simulink model "nonlinear_switch_intgr_mgntrqr_wndup_ctrl_closed_loop_sys"  (R2020b)
settings: Solver=VariableStepAuto  StartTime=0.0  StopTime=800  RelTol=1e-3
values from neighbouring files (symbols this model uses):
  COMMANDED_TORQUE_SATURATION = 0.05    [Workshop_MATLAB.m]
  COUPLING_COEFFICIENT = 0.5736    [Workshop_MATLAB.m]
  DEADZONE_REACTION_WHEEL_ANGULAR_MOMENTUM = REACTION_WHEEL_INERTIA * DEADZONE_REACTION_WHEEL_VELOCITY * dcgain(REACTION_WHEEL_ANGULAR_MOMENTUM.TRANSFER_FUNCTION)    [Workshop_MATLAB.m]
  deadzoneControllerGain = 0.1    [Workshop_MATLAB.m]
  DISTURBANCE_TORQUE = 0.001    [Workshop_MATLAB.m]
  DISTURBANCE_TORQUE_DELAY = 100    [Workshop_MATLAB.m]
  ESTIMATOR_TRANSFER_FUNCTION_DENOMINATOR = [ESTIMATOR_TIME_CONSTANT 1]    [Workshop_MATLAB.m]
  ESTIMATOR_TRANSFER_FUNCTION_NUMERATOR = [1 0]    [Workshop_MATLAB.m]
  FLEXIBLE_MODE_DAMPING_RATIO = 0.00495    [Workshop_MATLAB.m]
  FLEXIBLE_MODE_FREQUENCY = 2.6268    [Workshop_MATLAB.m]
  INITIAL_CONDITION_ON_STATE = 0.0001    [Workshop_MATLAB.m]
  MAGNETORQUER_CONTROLLER_GAIN = 0.001    [Workshop_MATLAB.m]
  MAXIMUM_LARGE_POINTING_ERROR = 25*2*pi/360    (= 0.436332312999)    [Workshop_MATLAB.m]
  MAXIMUM_TOLERABLE_POINTING_ERROR = 2.7*2*pi/360    (= 0.0471238898038)    [Workshop_MATLAB.m]
  MEASUREMENT_DELAY = 0.8    [Workshop_MATLAB.m]
  MEASUREMENT_NOISE_VARIANCE = 10^(-9)    (= 1e-09)    [Workshop_MATLAB.m]
  modalWithIntegratorGainMatrixStateFeedback = [0.0223 -0.55 -5.7]    [Workshop_MATLAB.m]
  NON_LINEAR_CONTROL_GAIN = 6    [Workshop_MATLAB.m]
  NON_LINEAR_CONTROL_SPEED_COMMAND = 0.15*pi/180    (= 0.00261799387799)    [Workshop_MATLAB.m]
  NON_LINEAR_CONTROL_SWITCHING_THRESHOLD = 3*pi/180    (= 0.0523598775598)    [Workshop_MATLAB.m]
  REACTION_WHEEL_DYNAMICS_DENOMINATOR = [1 2.400 0.763]    [Workshop_MATLAB.m]
  REACTION_WHEEL_DYNAMICS_NUMERATOR = REACTION_WHEEL_INERTIA*[1.214 0.763 0]    [Workshop_MATLAB.m]
  REACTION_WHEEL_INERTIA = 0.0004    [Workshop_MATLAB.m]
  REACTION_WHEEL_VELOCITY_SATURATION = 2800*2*pi/60    (= 293.215314335)    [Workshop_MATLAB.m]
  SATELLITE_INERTIA = 31.38    [Workshop_MATLAB.m]
  STAR_TRACKER_NOISE_DELAY = 160    [Workshop_MATLAB.m]
  UNLOADING_TORQUE_SATURATION = 0.0043    [Workshop_MATLAB.m]
undefined symbols (not defined in the file or in its folder): REACTION_WHEEL_ANGULAR_MOMENTUM, sigbuilder_block
libraries: dspsigops x2, simulink x1
settings Model: Creator=WLCG  LastModifiedBy=WLCG

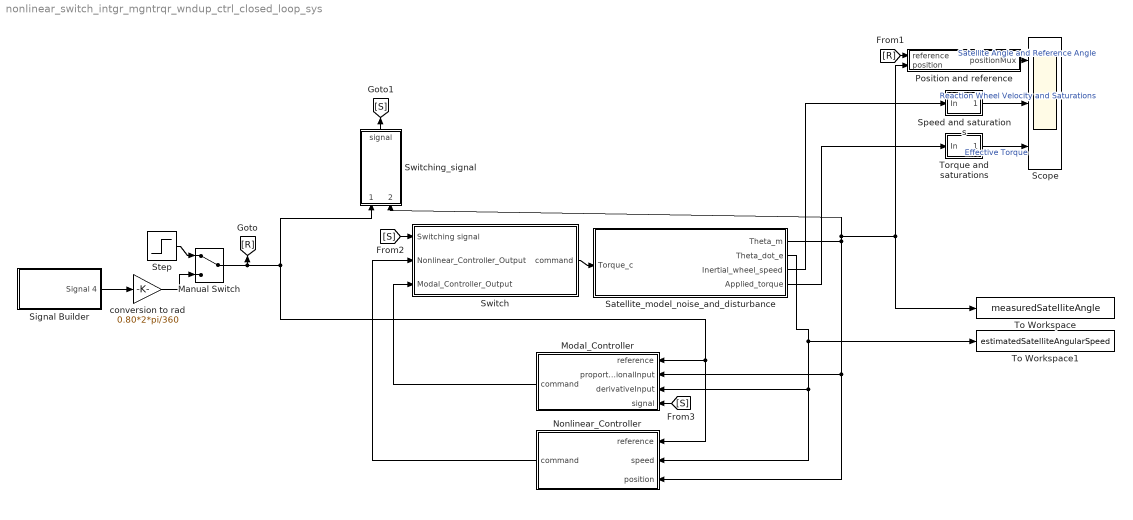
== system nonlinear_switch_intgr_mgntrqr_wndup_ctrl_closed_loop_sys ==
  Manual Switch : ManualSwitch
  Modal_Controller : Subsystem
  Nonlinear_Controller : Subsystem
  Position and reference : Subsystem
  Satellite_model_noise_and_disturbance : Subsystem
  Scope : Scope  NumInputPorts=3
  Signal Builder : Subsystem  Tag=STV Subsys  LoadFcn=sigbuilder_block('load');  StartFcn=sigbuilder_block('start');  StopFcn=sigbuilder_block('stop');  ClipboardFcn=sigbuilder_block('clipboard');  mask(Sigbuilder block){tuvar=[0:10]}
      mask help: Simulink:masks:SigbuilderBlock_MD
      mask init:
      | if ~strcmp(get_param(bdroot(gcbh),'SimulationStatus'),'stopped') tuvar = sigbuilder_block('maskInit'); end
      settings: CopyFcn=sigbuilder_block('copy');  DeleteFcn=sigbuilder_block('delete');  ModelCloseFcn=sigbuilder_block('modelClose');  PreSaveFcn=sigbuilder_block('preSave');  PauseFcn=sigbuilder_block('pause');  ContinueFcn=sigbuilder_block('continue');  NameChangeFcn=sigbuilder_block('namechange');  OpenFcn=sigbuilder_block('open',[371.25 48 550.5 359.25 ]);  CloseFcn=sigbuilder_block('close');
      mask Display: plot(0, 0, 100, 100,[2, 2, 32, 32, 2], [68, 8, 8, 68, 68],[32, 2], [38, 38], [32, 19, 2],[53, 60, 44], [32, 17, 17, 2],[16, 16, 31, 31]);txt = getActiveGroup(gcbh);text(2, 100, txt,'verticalAlignment', 'top');
  Speed and saturations : Subsystem
  Step : Step  Time=0  After=MAXIMUM_LARGE_POINTING_ERROR  SampleTime=0
  Switch : Subsystem
  Switching_signal : Subsystem
  To Workspace : ToWorkspace  VariableName=measuredSatelliteAngle  SaveFormat=Timeseries  SampleTime=-1
  To Workspace1 : ToWorkspace  VariableName=estimatedSatelliteAngularSpeed  SaveFormat=Timeseries  SampleTime=-1
  Torque and saturations : Subsystem
  conversion to rad : Gain  Gain=0.80*2*pi/360
  wires:
  Manual Switch/1 -> Switching_signal/1(reference), Nonlinear_Controller/1(reference), Modal_Controller/1(reference), [R]
  Satellite_model_noise_and_disturbance/1(Theta_m) -> Switching_signal/2(position), To Workspace/1, Position and reference/2(position), Nonlinear_Controller/3(position), Modal_Controller/2(proportionalInput)
  Position and reference/1(positionMux) -> Scope/1  "Satellite Angle and Reference Angle"
  Nonlinear_Controller/1(command) -> Switch/2(Nonlinear_Controller_Output)
  Modal_Controller/1(command) -> Switch/3(Modal_Controller_Output)
  Switch/1(command) -> Satellite_model_noise_and_disturbance/1(Torque_c)
  [R] -> Position and reference/1(reference)
  Satellite_model_noise_and_disturbance/2(Theta_dot_e) -> To Workspace1/1, Nonlinear_Controller/2(speed), Modal_Controller/3(derivativeInput)
  Satellite_model_noise_and_disturbance/3(Inertial_wheel_speed) -> Speed and saturations/1(In)
  Speed and saturations/1(Mux) -> Scope/2  "Reaction Wheel Velocity and Saturations"
  Satellite_model_noise_and_disturbance/4(Applied_torque) -> Torque and saturations/1(In)
  Torque and saturations/1(Mux) -> Scope/3  "Effective Torque"
  Switching_signal/1(signal) -> [S]
  [S] -> Switch/1(Switching signal)
  [S] -> Modal_Controller/4(signal)
  Step/1 -> Manual Switch/1
  Signal Builder/1(Signal 4) -> conversion to rad/1
  conversion to rad/1 -> Manual Switch/2

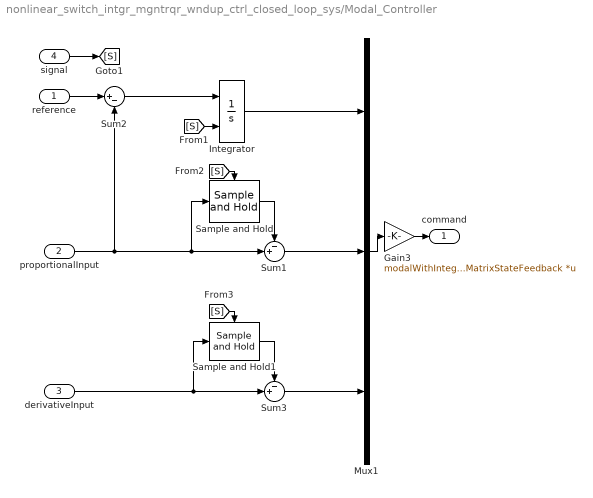
== system nonlinear_switch_intgr_mgntrqr_wndup_ctrl_closed_loop_sys/Modal_Controller ==
  reference : Inport
  proportionalInput : Inport  Port=2
  derivativeInput : Inport  Port=3
  signal : Inport  Port=4
  Gain3 : Gain  Gain=modalWithIntegratorGainMatrixStateFeedback  Multiplication=Matrix(K*u)
  Integrator : Integrator  ExternalReset=either
  Mux1 : Mux  Inputs=3
  Sample and Hold : dspsigops/Sample and Hold  trig=Either edge  initCond=0  latchinput=off
  Sample and Hold1 : dspsigops/Sample and Hold  trig=Either edge  initCond=0  latchinput=off
  Sum1 : Sum  Inputs=-+|
  Sum2 : Sum  Inputs=|+-
  Sum3 : Sum  Inputs=-+|
  command : Outport
  wires:
  Mux1/1 -> Gain3/1
  reference/1 -> Sum2/1
  Gain3/1 -> command/1
  Sum2/1 -> Integrator/1
  Integrator/1 -> Mux1/1
  proportionalInput/1 -> Sum2/2, Sample and Hold/1, Sum1/2
  Sum1/1 -> Mux1/2
  Sample and Hold/1 -> Sum1/1
  signal/1 -> [S]
  [S] -> Sample and Hold/Trigger
  [S] -> Integrator/2
  Sample and Hold1/1 -> Sum3/1
  [S] -> Sample and Hold1/Trigger
  derivativeInput/1 -> Sample and Hold1/1, Sum3/2
  Sum3/1 -> Mux1/3

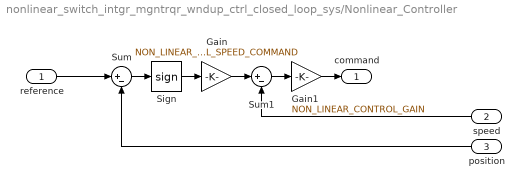
== system nonlinear_switch_intgr_mgntrqr_wndup_ctrl_closed_loop_sys/Nonlinear_Controller ==
  reference : Inport
  speed : Inport  Port=2
  position : Inport  Port=3
  Gain : Gain  Gain=NON_LINEAR_CONTROL_SPEED_COMMAND
  Gain1 : Gain  Gain=NON_LINEAR_CONTROL_GAIN
  Sign : Signum  ZeroCross=off
  Sum : Sum  Inputs=|+-
  Sum1 : Sum  Inputs=|+-
  command : Outport
  wires:
  reference/1 -> Sum/1
  Sum/1 -> Sign/1
  position/1 -> Sum/2
  Sign/1 -> Gain/1
  speed/1 -> Sum1/2
  Gain/1 -> Sum1/1
  Sum1/1 -> Gain1/1
  Gain1/1 -> command/1

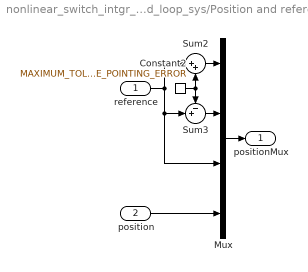
== system nonlinear_switch_intgr_mgntrqr_wndup_ctrl_closed_loop_sys/Position and reference ==
  reference : Inport
  position : Inport  Port=2
  Constant2 : Constant  Value=MAXIMUM_TOLERABLE_POINTING_ERROR
  Mux : Mux
  Sum2 : Sum  Inputs=|++
  Sum3 : Sum  Inputs=-+|
  positionMux : Outport
  wires:
  Constant2/1 -> Sum2/2, Sum3/1
  reference/1 -> Sum3/2, Mux/3, Sum2/1
  Sum3/1 -> Mux/2
  Sum2/1 -> Mux/1
  position/1 -> Mux/4
  Mux/1 -> positionMux/1

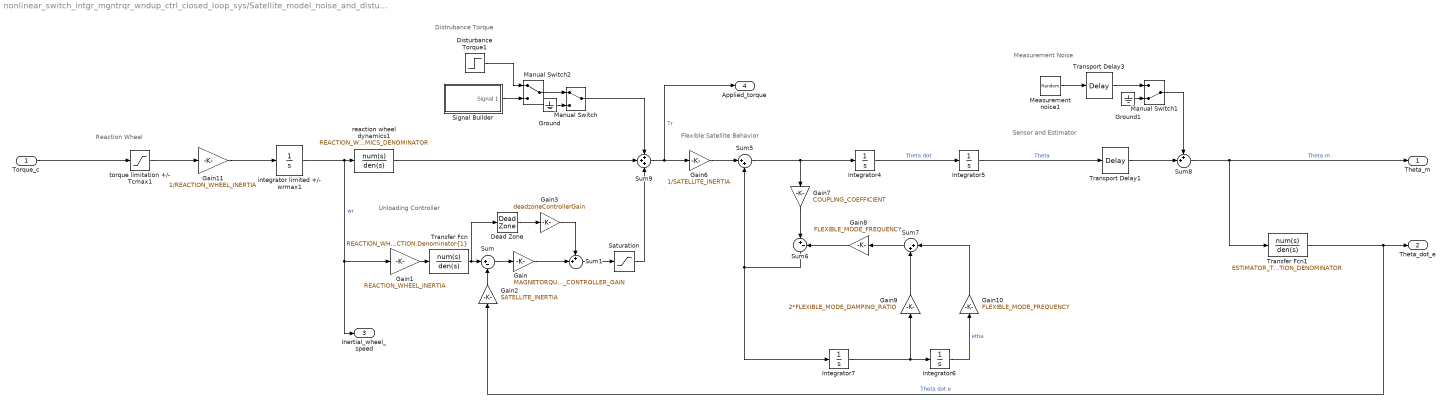
== system nonlinear_switch_intgr_mgntrqr_wndup_ctrl_closed_loop_sys/Satellite_model_noise_and_disturbance ==
  note: Unloading Controller
  note: Distrubance Torque
  note: Measurement Noise
  note: Sensor and Estimator
  note: Flexible Satellite Behavior
  note: Reaction Wheel
  Torque_c : Inport
  Dead Zone : DeadZone  LowerValue=-DEADZONE_REACTION_WHEEL_ANGULAR_MOMENTUM  UpperValue=DEADZONE_REACTION_WHEEL_ANGULAR_MOMENTUM  SaturateOnIntegerOverflow=on
  Disturbance Torque1 : Step  Time=DISTURBANCE_TORQUE_DELAY  After=DISTURBANCE_TORQUE  SampleTime=0
  Gain : Gain  Gain=MAGNETORQUER_CONTROLLER_GAIN
  Gain1 : Gain  Gain=REACTION_WHEEL_INERTIA
  Gain10 : Gain  Gain=FLEXIBLE_MODE_FREQUENCY
  Gain11 : Gain  Gain=1/REACTION_WHEEL_INERTIA
  Gain2 : Gain  Gain=SATELLITE_INERTIA
  Gain3 : Gain  Gain=deadzoneControllerGain
  Gain6 : Gain  Gain=1/SATELLITE_INERTIA
  Gain7 : Gain  Gain=COUPLING_COEFFICIENT
  Gain8 : Gain  Gain=FLEXIBLE_MODE_FREQUENCY
  Gain9 : Gain  Gain=2*FLEXIBLE_MODE_DAMPING_RATIO
  Ground : Ground
  Ground1 : Ground
  Integrator4 : Integrator
  Integrator5 : Integrator
  Integrator6 : Integrator  InitialCondition=INITIAL_CONDITION_ON_STATE
  Integrator7 : Integrator
  Manual Switch : ManualSwitch
  Manual Switch1 : ManualSwitch  CurrentSetting=0
  Manual Switch2 : ManualSwitch
  Measurement noice1 : RandomNumber  Variance=MEASUREMENT_NOISE_VARIANCE  SampleTime=0.01
  Saturation : Saturate  UpperLimit=UNLOADING_TORQUE_SATURATION  LowerLimit=-UNLOADING_TORQUE_SATURATION
  Signal Builder : Subsystem  Tag=STV Subsys  LoadFcn=sigbuilder_block('load');  StartFcn=sigbuilder_block('start');  StopFcn=sigbuilder_block('stop');  ClipboardFcn=sigbuilder_block('clipboard');  mask(Sigbuilder block){tuvar=[0:10]}
      mask help: Simulink:masks:SigbuilderBlock_MD
      mask init:
      | if ~strcmp(get_param(bdroot(gcbh),'SimulationStatus'),'stopped') tuvar = sigbuilder_block('maskInit'); end
      settings: CopyFcn=sigbuilder_block('copy');  DeleteFcn=sigbuilder_block('delete');  ModelCloseFcn=sigbuilder_block('modelClose');  PreSaveFcn=sigbuilder_block('preSave');  PauseFcn=sigbuilder_block('pause');  ContinueFcn=sigbuilder_block('continue');  NameChangeFcn=sigbuilder_block('namechange');  OpenFcn=sigbuilder_block('open',[322.5 150.75 550.5 359.25 ]);  CloseFcn=sigbuilder_block('close');
      mask Display: plot(0, 0, 100, 100,[2, 2, 32, 32, 2], [68, 8, 8, 68, 68],[32, 2], [38, 38], [32, 19, 2],[53, 60, 44], [32, 17, 17, 2],[16, 16, 31, 31]);txt = getActiveGroup(gcbh);text(2, 100, txt,'verticalAlignment', 'top');
  Sum : Sum  Inputs=|+-
  Sum1 : Sum  Inputs=++|
  Sum5 : Sum  Inputs=|++
  Sum6 : Sum  Inputs=|+-
  Sum7 : Sum  Inputs=|++
  Sum8 : Sum  Inputs=++|
  Sum9 : Sum  Inputs=+++
  Transfer Fcn : TransferFcn  Numerator=REACTION_WHEEL_ANGULAR_MOMENTUM.TRANSFER_FUNCTION.Numerator{1}  Denominator=REACTION_WHEEL_ANGULAR_MOMENTUM.TRANSFER_FUNCTION.Denominator{1}
  Transfer Fcn1 : TransferFcn  Numerator=ESTIMATOR_TRANSFER_FUNCTION_NUMERATOR  Denominator=ESTIMATOR_TRANSFER_FUNCTION_DENOMINATOR
  Transport Delay1 : TransportDelay  DelayTime=MEASUREMENT_DELAY
  Transport Delay3 : TransportDelay  DelayTime=STAR_TRACKER_NOISE_DELAY
  integrator limited +/- wrmax1 : Integrator  LimitOutput=on  UpperSaturationLimit=REACTION_WHEEL_VELOCITY_SATURATION  LowerSaturationLimit=-REACTION_WHEEL_VELOCITY_SATURATION
  reaction wheel dynamics1 : TransferFcn  Numerator=REACTION_WHEEL_DYNAMICS_NUMERATOR  Denominator=REACTION_WHEEL_DYNAMICS_DENOMINATOR
  torque limitation +/- Tcmax1 : Saturate  UpperLimit=COMMANDED_TORQUE_SATURATION  LowerLimit=-COMMANDED_TORQUE_SATURATION
  Theta_m : Outport
  Theta_dot_e : Outport  Port=2
  Inertial_wheel_speed : Outport  Port=3
  Applied_torque : Outport  Port=4
  wires:
  Signal Builder/1(Signal 1) -> Manual Switch2/2
  Gain6/1 -> Sum5/1
  Measurement noice1/1 -> Transport Delay3/1
  Gain9/1 -> Sum7/2
  Sum5/1 -> Gain7/1, Integrator4/1
  Gain7/1 -> Sum6/1
  torque limitation +/- Tcmax1/1 -> Gain11/1
  Sum8/1 -> Theta_m/1, Transfer Fcn1/1  "Theta m"
  Sum7/1 -> Gain8/1
  Integrator5/1 -> Transport Delay1/1  "Theta"
  Integrator6/1 -> Gain10/1  "etha"
  Torque_c/1 -> torque limitation +/- Tcmax1/1
  Integrator4/1 -> Integrator5/1  "Theta dot"
  Gain8/1 -> Sum6/2
  Integrator7/1 -> Integrator6/1, Gain9/1
  Sum9/1 -> Applied_torque/1, Gain6/1  "Tr"
  Transfer Fcn1/1 -> Gain2/1, Theta_dot_e/1  "Theta dot e"
  Sum6/1 -> Sum5/2, Integrator7/1
  reaction wheel dynamics1/1 -> Sum9/2
  Gain11/1 -> integrator limited +/- wrmax1/1
  Gain10/1 -> Sum7/1
  integrator limited +/- wrmax1/1 -> Gain1/1, Inertial_wheel_speed/1, reaction wheel dynamics1/1  "wr"
  Transport Delay1/1 -> Sum8/2
  Ground/1 -> Manual Switch/2
  Manual Switch/1 -> Sum9/1
  Ground1/1 -> Manual Switch1/2
  Manual Switch1/1 -> Sum8/1
  Transport Delay3/1 -> Manual Switch1/1
  Gain1/1 -> Transfer Fcn/1
  Transfer Fcn/1 -> Dead Zone/1, Sum/1
  Sum/1 -> Gain/1
  Gain2/1 -> Sum/2
  Dead Zone/1 -> Gain3/1
  Gain/1 -> Sum1/2
  Gain3/1 -> Sum1/1
  Sum1/1 -> Saturation/1
  Saturation/1 -> Sum9/3
  Disturbance Torque1/1 -> Manual Switch2/1
  Manual Switch2/1 -> Manual Switch/1

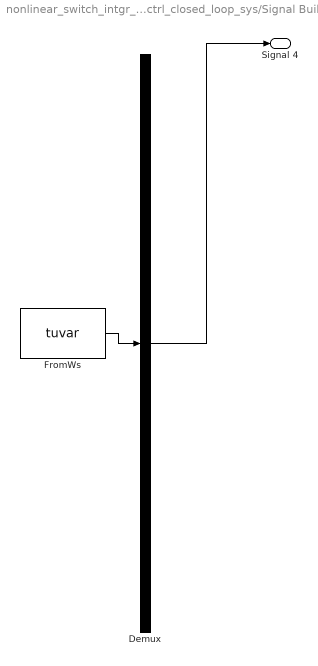
== system nonlinear_switch_intgr_mgntrqr_wndup_ctrl_closed_loop_sys/Signal Builder ==
  Demux : Demux  Tag=STV Demux  Outputs=1
      settings: DisplayOption=none
  FromWs : FromWorkspace  Tag=STV FromWs  VariableName=tuvar
      SigBuilderData=|
      | common.afterFinalStr = 'Extrapolate'
      | common.sampleTime = 0
      | dataSet.timeRange = [0 200]
      | dataSet.name = 'Group 1'
      | sbobj.Groups.Name = 'Group 1'
      | sbobj.Groups.Signals.Name = 'Signal 4'
      | sbobj.Groups.Signals.XData = [0 10 10 70 70 130 130 200]
      | sbobj.Groups.Signals.YData = [0 0 5 5 15 15 10 10]
      | sbobj.Groups.TimeRange = [0 200]
  Signal 4 : Outport  Tag=STV Outport
  wires:
  FromWs/1 -> Demux/1
  Demux/1 -> Signal 4/1

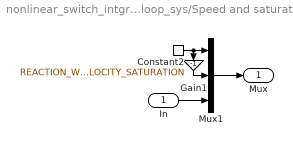
== system nonlinear_switch_intgr_mgntrqr_wndup_ctrl_closed_loop_sys/Speed and saturations ==
  In : Inport
  Constant2 : Constant  Value=REACTION_WHEEL_VELOCITY_SATURATION
  Gain1 : Gain  Gain=-1
  Mux1 : Mux  Inputs=3
  Mux : Outport
  wires:
  Gain1/1 -> Mux1/2
  In/1 -> Mux1/3
  Mux1/1 -> Mux/1
  Constant2/1 -> Gain1/1, Mux1/1

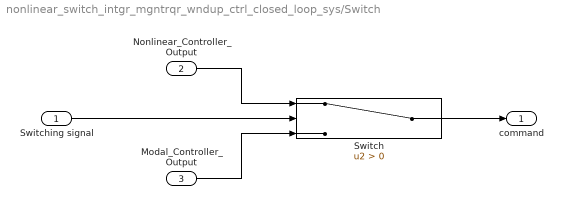
== system nonlinear_switch_intgr_mgntrqr_wndup_ctrl_closed_loop_sys/Switch ==
  Switching signal : Inport
  Nonlinear_Controller_Output : Inport  Port=2
  Modal_Controller_Output : Inport  Port=3
  Switch : Switch  Criteria=u2 > Threshold
  command : Outport
  wires:
  Modal_Controller_Output/1 -> Switch/3
  Nonlinear_Controller_Output/1 -> Switch/1
  Switch/1 -> command/1
  Switching signal/1 -> Switch/2

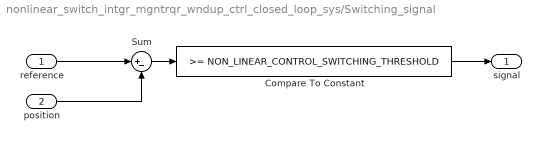
== system nonlinear_switch_intgr_mgntrqr_wndup_ctrl_closed_loop_sys/Switching_signal ==
  reference : Inport
  position : Inport  Port=2
  Compare To Constant : simulink/Logic and Bit Operations/Compare To Constant  relop=>=  const=NON_LINEAR_CONTROL_SWITCHING_THRESHOLD  OutDataTypeStr=boolean
  Sum : Sum  Inputs=|+-
  signal : Outport
  wires:
  reference/1 -> Sum/1
  Sum/1 -> Compare To Constant/1
  Compare To Constant/1 -> signal/1
  position/1 -> Sum/2

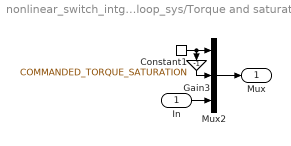
== system nonlinear_switch_intgr_mgntrqr_wndup_ctrl_closed_loop_sys/Torque and saturations ==
  In : Inport
  Constant1 : Constant  Value=COMMANDED_TORQUE_SATURATION
  Gain3 : Gain  Gain=-1
  Mux2 : Mux  Inputs=3
  Mux : Outport
  wires:
  Gain3/1 -> Mux2/2
  Mux2/1 -> Mux/1
  Constant1/1 -> Gain3/1, Mux2/1
  In/1 -> Mux2/3

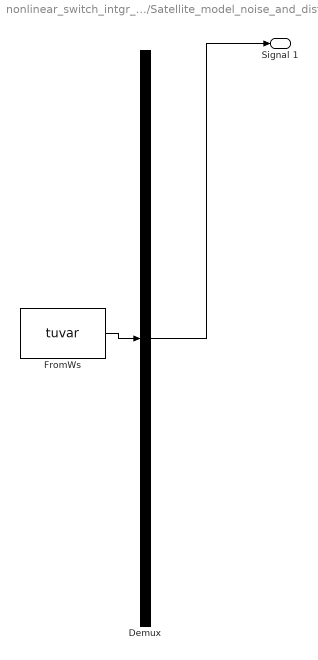
== system nonlinear_switch_intgr_mgntrqr_wndup_ctrl_closed_loop_sys/Satellite_model_noise_and_disturbance/Signal Builder ==
  Demux : Demux  Tag=STV Demux  Outputs=1
      settings: DisplayOption=none
  FromWs : FromWorkspace  Tag=STV FromWs  VariableName=tuvar
      SigBuilderData=|
      | common.afterFinalStr = 'Extrapolate'
      | common.sampleTime = 0
      | dataSet.timeRange = [0 800]
      | dataSet.name = 'Group 1'
      | sbobj.Groups.Name = 'Group 1'
      | sbobj.Groups.Signals.Name = 'Signal 1'
      | sbobj.Groups.Signals.XData = [0 200 200 500 500 800]
      | sbobj.Groups.Signals.YData = [0 0 0.001 0.001 0 0]
      | sbobj.Groups.TimeRange = [0 800]
  Signal 1 : Outport  Tag=STV Outport
  wires:
  FromWs/1 -> Demux/1
  Demux/1 -> Signal 1/1
